simulink model "SimulationEchantillinnesClampingMCC"  (R2017b)
settings: Solver=VariableStepAuto  StartTime=0.0  StopTime=Tf  MaxStep=Ts_elec  RelTol=1e-3
values from neighbouring files (symbols this model uses):
  C0 = 0.0    (= 0)    [DataMCCEchant.m]
  Cl = 0    [DataMCCEchant.m]
  F = 0.0001    [DataMCCEchant.m]
  Imax = Inom    (= 4.4)    [DataMCCEchant.m]
  Imin = 0    [DataMCCEchant.m]
  J = 2.20e-4    (= 0.00022)    [DataMCCEchant.m]
  Kelec = -place(Ae,Be,Pole_elec_desiree)    [DataMCCEchant.m]
  Kmeca = place(Am,Bm,Pole_meca_desiree)    [DataMCCEchant.m]
  Kphi = 0.061    [DataMCCEchant.m]
  L = 2.7e-3    (= 0.0027)    [DataMCCEchant.m]
  omref = 200    [DataMCCEchant.m]
  R = 1.22    [DataMCCEchant.m]
  Ts_elec = 1e-4    (= 0.0001)    [DataMCCEchant.m]
  Ts_meca = 100*Ts_elec    (= 0.01)    [DataMCCEchant.m]
  Vmax = Vdc    (= 24)    [DataMCCEchant.m]
  Vmin = 0    [DataMCCEchant.m]
undefined symbols (not defined in the file or in its folder): DiscIntNeverNeededParam
settings Model: Creator=romaindelpoux  LastModifiedBy=rdelpoux
settings SolverCC: ZeroCrossControl=DisableAll

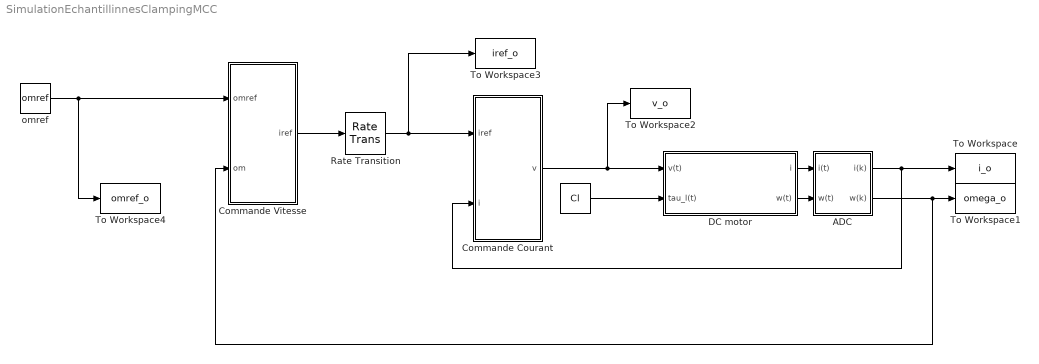
== system SimulationEchantillinnesClampingMCC ==
  " " : Constant  Value=Cl
  ADC : Subsystem
  Commande Courant : Subsystem
  Commande Vitesse : Subsystem
  DC motor : Subsystem
  Rate Transition : RateTransition  OutPortSampleTime=Ts_elec
  To Workspace : ToWorkspace  VariableName=i_o  SaveFormat=Timeseries  SampleTime=-1
  To Workspace1 : ToWorkspace  VariableName=omega_o  SaveFormat=Timeseries  SampleTime=-1
  To Workspace2 : ToWorkspace  VariableName=v_o  SaveFormat=Timeseries  SampleTime=-1
  To Workspace3 : ToWorkspace  VariableName=iref_o  SaveFormat=Timeseries  SampleTime=-1
  To Workspace4 : ToWorkspace  VariableName=omref_o  SaveFormat=Timeseries  SampleTime=-1
  omref : Constant  Value=omref
  wires:
  Commande Courant/1(v) -> To Workspace2/1, DC motor/1(v(t))
  omref/1 -> To Workspace4/1, Commande Vitesse/1(omref)
  Commande Vitesse/1(iref) -> Rate Transition/1
  " "/1 -> DC motor/2(tau_l(t))
  ADC/1(i(k)) -> Commande Courant/2(i), To Workspace/1
  ADC/2(w(k)) -> Commande Vitesse/2(om), To Workspace1/1
  DC motor/1(i) -> ADC/1(i(t))
  DC motor/2(w(t)) -> ADC/2(w(t))
  Rate Transition/1 -> To Workspace3/1, Commande Courant/1(iref)

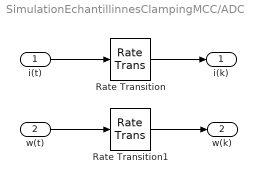
== system SimulationEchantillinnesClampingMCC/ADC ==
  i(t) : Inport
  w(t) : Inport  Port=2
  Rate Transition : RateTransition  OutPortSampleTime=Ts_elec
  Rate Transition1 : RateTransition  OutPortSampleTime=Ts_meca
  i(k) : Outport
  w(k) : Outport  Port=2
  wires:
  Rate Transition/1 -> i(k)/1
  Rate Transition1/1 -> w(k)/1
  i(t)/1 -> Rate Transition/1
  w(t)/1 -> Rate Transition1/1

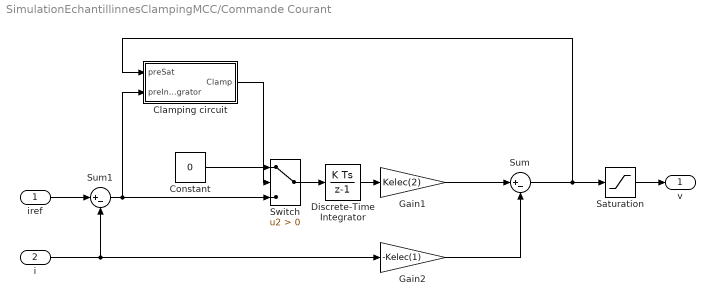
== system SimulationEchantillinnesClampingMCC/Commande Courant ==
  iref : Inport
  i : Inport  Port=2
  Clamping circuit : Subsystem
  Constant : Constant  Value=0
  Discrete-Time Integrator : DiscreteIntegrator  InitialConditionSetting=State (most efficient)  SampleTime=Ts_elec  ICPrevOutput=DiscIntNeverNeededParam  ICPrevScaledInput=DiscIntNeverNeededParam
  Gain1 : Gain  Gain=Kelec(2)
  Gain2 : Gain  Gain=-Kelec(1)
  Saturation : Saturate  UpperLimit=Vmax  LowerLimit=Vmin
  Sum : Sum  Inputs=|+-
  Sum1 : Sum  Inputs=|+-
  Switch : Switch  Criteria=u2 > Threshold  InputSameDT=on
  v : Outport
  wires:
  iref/1 -> Sum1/1
  i/1 -> Gain2/1, Sum1/2
  Discrete-Time Integrator/1 -> Gain1/1
  Gain1/1 -> Sum/1
  Gain2/1 -> Sum/2
  Constant/1 -> Switch/1
  Sum/1 -> Saturation/1, Clamping circuit/1(preSat)
  Sum1/1 -> Switch/3, Clamping circuit/2(preIntegrator)
  Saturation/1 -> v/1
  Switch/1 -> Discrete-Time Integrator/1
  Clamping circuit/1(Clamp) -> Switch/2

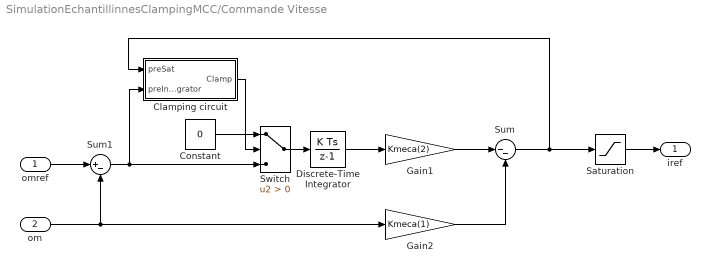
== system SimulationEchantillinnesClampingMCC/Commande Vitesse ==
  omref : Inport
  om : Inport  Port=2
  Clamping circuit : Subsystem
  Constant : Constant  Value=0
  Discrete-Time Integrator : DiscreteIntegrator  InitialConditionSetting=State (most efficient)  SampleTime=Ts_meca  ICPrevOutput=DiscIntNeverNeededParam  ICPrevScaledInput=DiscIntNeverNeededParam
  Gain1 : Gain  Gain=Kmeca(2)
  Gain2 : Gain  Gain=Kmeca(1)
  Saturation : Saturate  UpperLimit=Imax  LowerLimit=Imin
  Sum : Sum  Inputs=|--
  Sum1 : Sum  Inputs=|+-
  Switch : Switch  Criteria=u2 > Threshold  InputSameDT=on
  iref : Outport
  wires:
  Gain1/1 -> Sum/1
  Discrete-Time Integrator/1 -> Gain1/1
  omref/1 -> Sum1/1
  Gain2/1 -> Sum/2
  om/1 -> Gain2/1, Sum1/2
  Sum/1 -> Clamping circuit/1(preSat), Saturation/1
  Saturation/1 -> iref/1
  Switch/1 -> Discrete-Time Integrator/1
  Sum1/1 -> Switch/3, Clamping circuit/2(preIntegrator)
  Clamping circuit/1(Clamp) -> Switch/2
  Constant/1 -> Switch/1

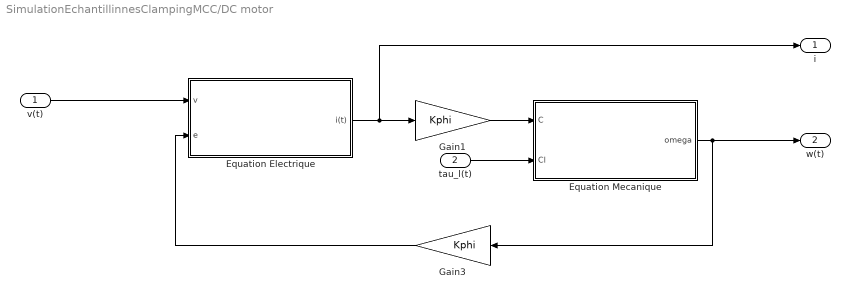
== system SimulationEchantillinnesClampingMCC/DC motor ==
  v(t) : Inport
  tau_l(t) : Inport  Port=2
  Equation Electrique : Subsystem
  Equation Mecanique : Subsystem
  Gain1 : Gain  Gain=Kphi
  "Gain3  " : Gain  Gain=Kphi
  i : Outport
  w(t) : Outport  Port=2
  wires:
  "Gain3  "/1 -> Equation Electrique/2(e)
  Gain1/1 -> Equation Mecanique/1(C)
  tau_l(t)/1 -> Equation Mecanique/2(Cl)
  Equation Electrique/1(i(t)) -> i/1, Gain1/1
  Equation Mecanique/1(omega) -> w(t)/1, "Gain3  "/1
  v(t)/1 -> Equation Electrique/1(v)

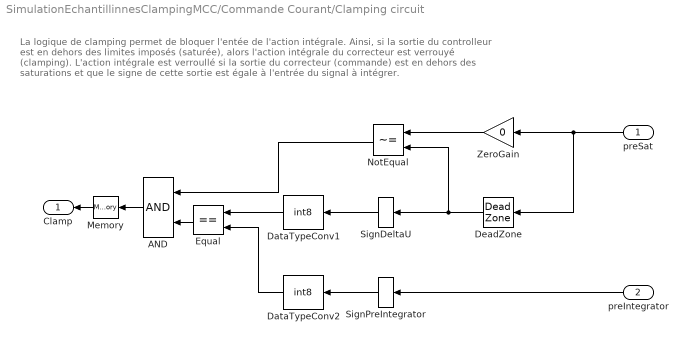
== system SimulationEchantillinnesClampingMCC/Commande Courant/Clamping circuit ==
  note: La logique de clamping permet de bloquer l'entée de l'action intégrale.
      | Ainsi, si la sortie du controlleur est en dehors des limites imposés (saturée), alors l'action intégrale du correcteur est verrouyé (clamping).
      | L'action intégrale est verroullé si la sortie du correcteur (commande) est en dehors des saturations et que le signe de cette sortie est égale
      | à l'entrée du signal à intégrer.
  preSat : Inport  DisableCoverage=on
  preIntegrator : Inport  DisableCoverage=on  Port=2
  AND : Logic  DisableCoverage=on
  DataTypeConv1 : DataTypeConversion  DisableCoverage=on  OutDataTypeStr=int8  SaturateOnIntegerOverflow=on  RndMeth=Zero  LockScale=on
  DataTypeConv2 : DataTypeConversion  DisableCoverage=on  OutDataTypeStr=int8
  DeadZone : DeadZone  DisableCoverage=on  LowerValue=Vmin  UpperValue=Vmax
  Equal : RelationalOperator  DisableCoverage=on  Operator===  RndMeth=Nearest  InputSameDT=on
  Memory : Memory  DisableCoverage=on
  NotEqual : RelationalOperator  DisableCoverage=on  Operator=~=  RndMeth=Nearest  InputSameDT=on
  SignDeltaU : Signum  DisableCoverage=on
  SignPreIntegrator : Signum  DisableCoverage=on
  ZeroGain : Gain  DisableCoverage=on  Gain=0  SaturateOnIntegerOverflow=on  OutDataTypeStr=Inherit: Same as input  ParamDataTypeStr=Inherit: Same as input
  Clamp : Outport  DisableCoverage=on
  wires:
  preSat/1 -> ZeroGain/1, DeadZone/1
  preIntegrator/1 -> SignPreIntegrator/1
  ZeroGain/1 -> NotEqual/1
  DeadZone/1 -> NotEqual/2, SignDeltaU/1
  SignDeltaU/1 -> DataTypeConv1/1
  DataTypeConv1/1 -> Equal/1
  SignPreIntegrator/1 -> DataTypeConv2/1
  DataTypeConv2/1 -> Equal/2
  NotEqual/1 -> AND/1
  Equal/1 -> AND/2
  AND/1 -> Memory/1
  Memory/1 -> Clamp/1

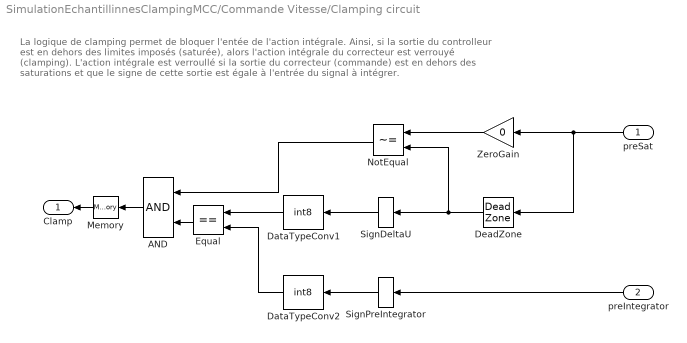
== system SimulationEchantillinnesClampingMCC/Commande Vitesse/Clamping circuit ==
  note: La logique de clamping permet de bloquer l'entée de l'action intégrale.
      | Ainsi, si la sortie du controlleur est en dehors des limites imposés (saturée), alors l'action intégrale du correcteur est verrouyé (clamping).
      | L'action intégrale est verroullé si la sortie du correcteur (commande) est en dehors des saturations et que le signe de cette sortie est égale
      | à l'entrée du signal à intégrer.
  preSat : Inport  DisableCoverage=on
  preIntegrator : Inport  DisableCoverage=on  Port=2
  AND : Logic  DisableCoverage=on
  DataTypeConv1 : DataTypeConversion  DisableCoverage=on  OutDataTypeStr=int8  SaturateOnIntegerOverflow=on  RndMeth=Zero  LockScale=on
  DataTypeConv2 : DataTypeConversion  DisableCoverage=on  OutDataTypeStr=int8
  DeadZone : DeadZone  DisableCoverage=on  LowerValue=Imin  UpperValue=Imax
  Equal : RelationalOperator  DisableCoverage=on  Operator===  RndMeth=Nearest  InputSameDT=on
  Memory : Memory  DisableCoverage=on
  NotEqual : RelationalOperator  DisableCoverage=on  Operator=~=  RndMeth=Nearest  InputSameDT=on
  SignDeltaU : Signum  DisableCoverage=on
  SignPreIntegrator : Signum  DisableCoverage=on
  ZeroGain : Gain  DisableCoverage=on  Gain=0  SaturateOnIntegerOverflow=on  OutDataTypeStr=Inherit: Same as input  ParamDataTypeStr=Inherit: Same as input
  Clamp : Outport  DisableCoverage=on
  wires:
  preSat/1 -> ZeroGain/1, DeadZone/1
  preIntegrator/1 -> SignPreIntegrator/1
  ZeroGain/1 -> NotEqual/1
  DeadZone/1 -> NotEqual/2, SignDeltaU/1
  SignDeltaU/1 -> DataTypeConv1/1
  DataTypeConv1/1 -> Equal/1
  SignPreIntegrator/1 -> DataTypeConv2/1
  DataTypeConv2/1 -> Equal/2
  NotEqual/1 -> AND/1
  Equal/1 -> AND/2
  AND/1 -> Memory/1
  Memory/1 -> Clamp/1

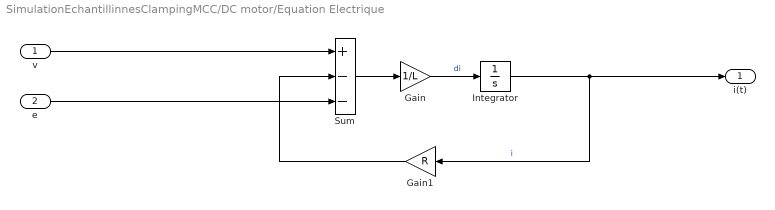
== system SimulationEchantillinnesClampingMCC/DC motor/Equation Electrique ==
  v : Inport
  e : Inport  Port=2
  Gain : Gain  Gain=1/L
  Gain1 : Gain  Gain=R
  Integrator : Integrator
  Sum : Sum  Inputs=+--
  i(t) : Outport
  wires:
  Gain1/1 -> Sum/2
  Sum/1 -> Gain/1
  Integrator/1 -> i(t)/1, Gain1/1  "i"
  Gain/1 -> Integrator/1  "di"
  v/1 -> Sum/1
  e/1 -> Sum/3

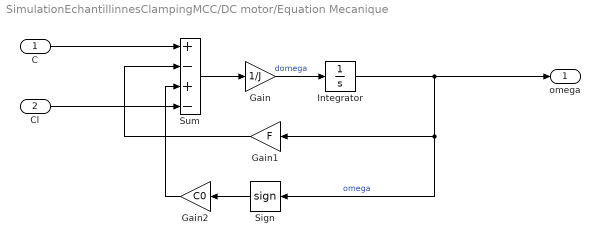
== system SimulationEchantillinnesClampingMCC/DC motor/Equation Mecanique ==
  C : Inport
  Cl : Inport  Port=2
  Gain : Gain  Gain=1/J
  Gain1 : Gain  Gain=F
  Gain2 : Gain  Gain=C0
  Integrator : Integrator
  Sign : Signum
  Sum : Sum  Inputs=+-+-
  omega : Outport
  wires:
  Gain/1 -> Integrator/1  "domega"
  Integrator/1 -> Sign/1, Gain1/1, omega/1  "omega"
  Sum/1 -> Gain/1
  Gain1/1 -> Sum/2
  Sign/1 -> Gain2/1
  Gain2/1 -> Sum/3
  C/1 -> Sum/1
  Cl/1 -> Sum/4
